simulink model "CtrPlatform_AdaptiveControl"  (Simulink 7.9)
settings: Solver=ode3  StartTime=0.0  StopTime=8  FixedStep=Ts  RelTol=1e-3
InitFcn:
  | eval('CtrPlatformCfg')
StopFcn:
  | eval('CtrPlotTrj')
values from neighbouring files (symbols this model uses):
  A = [a1 a2 a3 a4 a5 a6]/180*pi    [Config.m]    (also in CtrPlatformCfg.m)
  a2 = 0    [Config.m]    (also in CtrPlatformCfg.m)
  a3 = 0    [Config.m]    (also in CtrPlatformCfg.m)
  a4 = 0    [Config.m]    (also in CtrPlatformCfg.m)
  a5 = 90    [Config.m]    (also in CtrPlatformCfg.m)
  a6 = 0    [Config.m]    (also in CtrPlatformCfg.m)
  Cen = Cen(:)'    [Config.m]    (also in CtrPlatformCfg.m; DynEulerTest.m = Cen'; EfDynCAD.m = [cen1,cen2,cen3,cen4,cen5,cen6]')
  CurPulseFreq = 0.25*2*pi    (= 1.57079632679)    [Config.m]    (also in CtrPlatformCfg.m)
  Deg2Rad = pi/180    (= 0.0174532925199)    [Config.m]    (also in CtrPlatformCfg.m)
  DisturbSelect = 2    [Config.m]    (also in CtrPlatformCfg.m)
  DynTrjMode = 3    [Config.m]    (also in CtrPlatformCfg.m = 1)
  FbDisturbSelect = 2    [Config.m]    (also in CtrPlatformCfg.m)
  freq = tvel/radius    (= 1)    [Config.m]    (also in CtrPlatformCfg.m)
  FrictionSelect = 2    [CtrPlatformCfg.m]
  Gravity = 9.8    [Config.m]    (also in CtrPlatformCfg.m)
  Ie1 = in1(:)'    [Config.m]    (also in CtrPlatformCfg.m; DynEulerTest.m = in1(:); EfDynCAD.m = in1(:))
  Ie2 = in2(:)'    [Config.m]    (also in CtrPlatformCfg.m; DynEulerTest.m = in2(:); EfDynCAD.m = in2(:))
  Ie3 = in3(:)'    [Config.m]    (also in CtrPlatformCfg.m; DynEulerTest.m = in3(:); EfDynCAD.m = in3(:))
  Ie4 = in4(:)'    [Config.m]    (also in CtrPlatformCfg.m; DynEulerTest.m = in4(:); EfDynCAD.m = in4(:))
  Ie5 = in5(:)'    [Config.m]    (also in CtrPlatformCfg.m; DynEulerTest.m = in5(:); EfDynCAD.m = in5(:))
  Ie6 = in6(:)'    [Config.m]    (also in CtrPlatformCfg.m; DynEulerTest.m = in6(:); EfDynCAD.m = in6(:))
  in1 = [5.2954 -0.2565 -0.6366;-0.2565 4.7000 0.2830;-0.6366 0.2829 5.8635]    [Config.m]    (also in CtrPlatformCfg.m; DynEulerTest.m; EfDynCAD.m = [0.54  -0.01 0.23)
  in2 = [5.8840 0.0072 0.0135;0.0072 6.0178 -0.1907;0.0135 -0.1907 0.3374]    [Config.m]    (also in CtrPlatformCfg.m; DynEulerTest.m; EfDynCAD.m = (R_x*R_z)*in2*(R_x*R_z)')
  in3 = [1.8201 -0.2274 -0.3112;-0.2274 2.2537 -0.1441;-0.3112 -0.1441 1.9485]    [Config.m]    (also in CtrPlatformCfg.m; DynEulerTest.m; EfDynCAD.m = (R_x*R_z)*in3*(R_x*R_z)')
  in4 = [0.0607 -0.0922 0;-0.0922 1.4493 0;0 0 1.4620]    [Config.m]    (also in CtrPlatformCfg.m; DynEulerTest.m = [0.0607 -0.0922 0;-0.0922 1.4493 0;0 0,1.4620]; EfDynCAD.m = (R_y*Rz)*in4*(R_y*Rz)')
  in5 = [0.0191 0.0032 0;0.0032 0.0228 0;0 0 0.0291]    [Config.m]    (also in CtrPlatformCfg.m; DynEulerTest.m; EfDynCAD.m = (R_x*R_y)*in5*(R_x*R_y)')
  in6 = [0.0012 0 0;0 0.0007 0;0 0 0.0007]    [Config.m]    (also in CtrPlatformCfg.m; DynEulerTest.m; EfDynCAD.m = (R_y*Rz)*in6*(R_y*Rz)')
  init_Endx = gd_init(1,4)    [Config.m]    (also in CtrPlatformCfg.m)
  init_Endy = gd_init(2,4)    [Config.m]    (also in CtrPlatformCfg.m)
  init_Endz = gd_init(3,4)    [Config.m]    (also in CtrPlatformCfg.m)
  init_Rot = gd_init(1:3,1:3)    [Config.m]    (also in CtrPlatformCfg.m)
  InitialPos1 = A(1)*Rad2Line(1)    [CtrPlatformCfg.m]
  InitialPos2 = A(2)*Rad2Line(2)    [CtrPlatformCfg.m]
  InitialPos3 = A(3)*Rad2Line(3)    [CtrPlatformCfg.m]
  InitialPos4 = A(4)*Rad2Line(4)    [CtrPlatformCfg.m]
  InitialPos5 = A(5)*Rad2Line(5)    [CtrPlatformCfg.m]
  InitialPos6 = A(6)*Rad2Line(6)    [CtrPlatformCfg.m]
  JntOffset1 = A(1)    [Config.m]    (also in CtrPlatformCfg.m)
  JntOffset2 = A(2)    [Config.m]    (also in CtrPlatformCfg.m)
  JntOffset3 = A(3)    [Config.m]    (also in CtrPlatformCfg.m)
  JntOffset4 = A(4)    [Config.m]    (also in CtrPlatformCfg.m)
  JntOffset5 = A(5)    [Config.m]    (also in CtrPlatformCfg.m)
  JntOffset6 = A(6)    [Config.m]    (also in CtrPlatformCfg.m)
  L = [l1 l2 l3 l4 l5 l6 l7 l8 l9]    [Config.m]    (also in CtrPlatformCfg.m)
  LinePTs2RadpS = 2*pi/(EncRes*Ts)./Gear    [Config.m]    (also in CtrPlatformCfg.m)
  LinePTs2Rpm = 60/(EncRes*Ts)    (= 7.32421875)    [Config.m]    (also in CtrPlatformCfg.m)
  Ma = [ma1 ma2 ma3 ma4 ma5 ma6]    [Config.m]    (also in CtrPlatformCfg.m; DynEulerTest.m = [ma1; ma2; ma3; ma4; ma5; ma6]; EfDynCAD.m = [ma1 ma2 ma3 ma4 ma5 ma6]')
  ma1 = 170.31    [Config.m]    (also in CtrPlatformCfg.m; DynEulerTest.m; EfDynCAD.m = 77.75)
  ma2 = 63.74    [Config.m]    (also in CtrPlatformCfg.m; DynEulerTest.m; EfDynCAD.m = 32.31)
  ma3 = 98.98    [Config.m]    (also in CtrPlatformCfg.m; DynEulerTest.m; EfDynCAD.m = 18.61)
  ma4 = 24.46    [Config.m]    (also in CtrPlatformCfg.m; DynEulerTest.m; EfDynCAD.m = 15.65)
  ma5 = 5.24    [Config.m]    (also in CtrPlatformCfg.m; DynEulerTest.m; EfDynCAD.m = 3.32)
  ma6 = 0.6    [Config.m]    (also in CtrPlatformCfg.m; DynEulerTest.m; EfDynCAD.m)
  Pi0 = PiTest    [CtrPlatformCfg.m]
  PosPulseEnable = 1    [Config.m]    (also in CtrPlatformCfg.m)
  PosSourceSelect_Ad = 2    [CtrPlatformCfg.m]
  PosVelPulseGain = 500    [Config.m]    (also in CtrPlatformCfg.m)
  Rad2Line = Gear*EncRes/(2*pi)    [Config.m]    (also in CtrPlatformCfg.m)
  Rpm2LinePTs = EncRes*Ts/60    (= 0.136533333333)    [Config.m]    (also in CtrPlatformCfg.m)
  TrajSwitch = 1    [Config.m]    (also in CtrPlatformCfg.m)
  Trq2Cur = Trq2Cur./Cur2Trq    [Config.m]    (also in CtrPlatformCfg.m)
  Ts = 1/FrHz    (= 0.00025)    [Config.m]    (also in CtrPlatformCfg.m)
  Ts_Dyn = Ts    (= 0.00025)    [Config.m]    (also in CtrPlatformCfg.m)
  tvel = 120    [Config.m]    (also in CtrPlatformCfg.m)
  VelLpAxisNum = 1    [Config.m]    (also in CtrPlatformCfg.m)
  VelPulseEnable = 0    [Config.m]    (also in CtrPlatformCfg.m)
  VelPulseGain = 500    [Config.m]    (also in CtrPlatformCfg.m)
  Volt2Trq = Volt2Trq./Trq2Cur    [Config.m]    (also in CtrPlatformCfg.m)
undefined symbols (not defined in the file or in its folder): a1, DiscIntNeverNeededParam
libraries: simulink x56, mblibv1 x35, powerlib_extras x8, commnoisgen2 x2
(part 4 of 4)

== system CtrPlatform_AdaptiveControl/Friction Torque/Friction Torque/Ff2/Fp ==
  q : Inport
  Add : Sum  Inputs=++++  SampleTime=Ts
  B1 : Gain  Gain=B1  SampleTime=Ts
  B2 : Gain  Gain=B2  SampleTime=Ts
  B3 : Gain  Gain=B3  SampleTime=Ts
  B4 : Gain  Gain=B4  SampleTime=Ts
  Cosine : simulink/Lookup Tables/Cosine  Formula=cos(2*pi*u)  NumDataPoints=(2^5)+1  OutputWordLength=16
  Cosine1 : simulink/Lookup Tables/Cosine  Formula=cos(2*pi*u)  NumDataPoints=(2^5)+1  OutputWordLength=16
  Gain : Gain  Gain=1/(2*pi)  SampleTime=Ts
  Gain1 : Gain  Gain=1/pi  SampleTime=Ts
  Sine : simulink/Lookup Tables/Sine  Formula=sin(2*pi*u)  NumDataPoints=(2^5)+1  OutputWordLength=16
  Sine1 : simulink/Lookup Tables/Sine  Formula=sin(2*pi*u)  NumDataPoints=(2^5)+1  OutputWordLength=16
  Fp : Outport
  wires:
  Gain/1 -> Sine/1, Cosine/1
  Gain1/1 -> Sine1/1, Cosine1/1
  q/1 -> Gain/1, Gain1/1
  Cosine1/1 -> B4/1
  Sine1/1 -> B3/1
  Cosine/1 -> B2/1
  Sine/1 -> B1/1
  B2/1 -> Add/2
  B3/1 -> Add/3
  B4/1 -> Add/4
  B1/1 -> Add/1
  Add/1 -> Fp/1

== system CtrPlatform_AdaptiveControl/Friction Torque/Friction Torque/Ff2/Fv ==
  dq : Inport
  Abs : Abs  SampleTime=Ts
  Add : Sum  SampleTime=Ts
  Add1 : Sum  SampleTime=Ts
  Divide : Product  Inputs=*/  SampleTime=Ts
  Gain : Constant  Value=-1  SampleTime=Ts
  Math Function : Math  Operator=pow  SampleTime=Ts  SaturateOnIntegerOverflow=on
  Math Function1 : Math  SampleTime=Ts  SaturateOnIntegerOverflow=on
  Product{,1..3} (4 alike) : Product  SampleTime=Ts  RndMeth=Zero
  Sign : Signum  SampleTime=Ts
  Subtract : Sum  Inputs=-+  SampleTime=Ts
  dqs : Constant  Value=dqs  SampleTime=Ts
  fc : Constant  Value=fc  SampleTime=Ts
  fs : Constant  Value=fs  SampleTime=Ts
  lamda : Constant  Value=lamda  SampleTime=Ts
  theta : Constant  Value=theta  SampleTime=Ts
  Fv : Outport
  wires:
  dq/1 -> Divide/1, Sign/1, Product3/2
  dqs/1 -> Divide/2
  Divide/1 -> Abs/1
  Abs/1 -> Math Function/1
  lamda/1 -> Math Function/2
  Math Function/1 -> Product/1
  Gain/1 -> Product/2
  Product/1 -> Math Function1/1
  fc/1 -> Subtract/1, Add/1
  fs/1 -> Subtract/2
  Subtract/1 -> Product1/1
  Math Function1/1 -> Product1/2
  Product1/1 -> Add/2
  Sign/1 -> Product2/1
  Add/1 -> Product2/2
  Product3/1 -> Add1/1
  Product2/1 -> Add1/2
  theta/1 -> Product3/1
  Add1/1 -> Fv/1

== system CtrPlatform_AdaptiveControl/Friction Torque/Friction Torque/Ff3/Fp ==
  q : Inport
  Add : Sum  Inputs=++++  SampleTime=Ts
  B1 : Gain  Gain=B1  SampleTime=Ts
  B2 : Gain  Gain=B2  SampleTime=Ts
  B3 : Gain  Gain=B3  SampleTime=Ts
  B4 : Gain  Gain=B4  SampleTime=Ts
  Cosine : simulink/Lookup Tables/Cosine  Formula=cos(2*pi*u)  NumDataPoints=(2^5)+1  OutputWordLength=16
  Cosine1 : simulink/Lookup Tables/Cosine  Formula=cos(2*pi*u)  NumDataPoints=(2^5)+1  OutputWordLength=16
  Gain : Gain  Gain=1/(2*pi)  SampleTime=Ts
  Gain1 : Gain  Gain=1/pi  SampleTime=Ts
  Sine : simulink/Lookup Tables/Sine  Formula=sin(2*pi*u)  NumDataPoints=(2^5)+1  OutputWordLength=16
  Sine1 : simulink/Lookup Tables/Sine  Formula=sin(2*pi*u)  NumDataPoints=(2^5)+1  OutputWordLength=16
  Fp : Outport
  wires:
  Gain/1 -> Sine/1, Cosine/1
  Gain1/1 -> Sine1/1, Cosine1/1
  q/1 -> Gain/1, Gain1/1
  Cosine1/1 -> B4/1
  Sine1/1 -> B3/1
  Cosine/1 -> B2/1
  Sine/1 -> B1/1
  B2/1 -> Add/2
  B3/1 -> Add/3
  B4/1 -> Add/4
  B1/1 -> Add/1
  Add/1 -> Fp/1

== system CtrPlatform_AdaptiveControl/Friction Torque/Friction Torque/Ff3/Fv ==
  dq : Inport
  Abs : Abs  SampleTime=Ts
  Add : Sum  SampleTime=Ts
  Add1 : Sum  SampleTime=Ts
  Divide : Product  Inputs=*/  SampleTime=Ts
  Gain : Constant  Value=-1  SampleTime=Ts
  Math Function : Math  Operator=pow  SampleTime=Ts  SaturateOnIntegerOverflow=on
  Math Function1 : Math  SampleTime=Ts  SaturateOnIntegerOverflow=on
  Product{,1..3} (4 alike) : Product  SampleTime=Ts  RndMeth=Zero
  Sign : Signum  SampleTime=Ts
  Subtract : Sum  Inputs=-+  SampleTime=Ts
  dqs : Constant  Value=dqs  SampleTime=Ts
  fc : Constant  Value=fc  SampleTime=Ts
  fs : Constant  Value=fs  SampleTime=Ts
  lamda : Constant  Value=lamda  SampleTime=Ts
  theta : Constant  Value=theta  SampleTime=Ts
  Fv : Outport
  wires:
  dq/1 -> Divide/1, Sign/1, Product3/2
  dqs/1 -> Divide/2
  Divide/1 -> Abs/1
  Abs/1 -> Math Function/1
  lamda/1 -> Math Function/2
  Math Function/1 -> Product/1
  Gain/1 -> Product/2
  Product/1 -> Math Function1/1
  fc/1 -> Subtract/1, Add/1
  fs/1 -> Subtract/2
  Subtract/1 -> Product1/1
  Math Function1/1 -> Product1/2
  Product1/1 -> Add/2
  Sign/1 -> Product2/1
  Add/1 -> Product2/2
  Product3/1 -> Add1/1
  Product2/1 -> Add1/2
  theta/1 -> Product3/1
  Add1/1 -> Fv/1

== system CtrPlatform_AdaptiveControl/Friction Torque/Friction Torque/Ff4/Fp ==
  q : Inport
  Add : Sum  Inputs=++++  SampleTime=Ts
  B1 : Gain  Gain=B1  SampleTime=Ts
  B2 : Gain  Gain=B2  SampleTime=Ts
  B3 : Gain  Gain=B3  SampleTime=Ts
  B4 : Gain  Gain=B4  SampleTime=Ts
  Cosine : simulink/Lookup Tables/Cosine  Formula=cos(2*pi*u)  NumDataPoints=(2^5)+1  OutputWordLength=16
  Cosine1 : simulink/Lookup Tables/Cosine  Formula=cos(2*pi*u)  NumDataPoints=(2^5)+1  OutputWordLength=16
  Gain : Gain  Gain=1/(2*pi)  SampleTime=Ts
  Gain1 : Gain  Gain=1/pi  SampleTime=Ts
  Sine : simulink/Lookup Tables/Sine  Formula=sin(2*pi*u)  NumDataPoints=(2^5)+1  OutputWordLength=16
  Sine1 : simulink/Lookup Tables/Sine  Formula=sin(2*pi*u)  NumDataPoints=(2^5)+1  OutputWordLength=16
  Fp : Outport
  wires:
  Gain/1 -> Sine/1, Cosine/1
  Gain1/1 -> Sine1/1, Cosine1/1
  q/1 -> Gain/1, Gain1/1
  Cosine1/1 -> B4/1
  Sine1/1 -> B3/1
  Cosine/1 -> B2/1
  Sine/1 -> B1/1
  B2/1 -> Add/2
  B3/1 -> Add/3
  B4/1 -> Add/4
  B1/1 -> Add/1
  Add/1 -> Fp/1

== system CtrPlatform_AdaptiveControl/Friction Torque/Friction Torque/Ff4/Fv ==
  dq : Inport
  Abs : Abs  SampleTime=Ts
  Add : Sum  SampleTime=Ts
  Add1 : Sum  SampleTime=Ts
  Divide : Product  Inputs=*/  SampleTime=Ts
  Gain : Constant  Value=-1  SampleTime=Ts
  Math Function : Math  Operator=pow  SampleTime=Ts  SaturateOnIntegerOverflow=on
  Math Function1 : Math  SampleTime=Ts  SaturateOnIntegerOverflow=on
  Product{,1..3} (4 alike) : Product  SampleTime=Ts  RndMeth=Zero
  Sign : Signum  SampleTime=Ts
  Subtract : Sum  Inputs=-+  SampleTime=Ts
  dqs : Constant  Value=dqs  SampleTime=Ts
  fc : Constant  Value=fc  SampleTime=Ts
  fs : Constant  Value=fs  SampleTime=Ts
  lamda : Constant  Value=lamda  SampleTime=Ts
  theta : Constant  Value=theta  SampleTime=Ts
  Fv : Outport
  wires:
  dq/1 -> Divide/1, Sign/1, Product3/2
  dqs/1 -> Divide/2
  Divide/1 -> Abs/1
  Abs/1 -> Math Function/1
  lamda/1 -> Math Function/2
  Math Function/1 -> Product/1
  Gain/1 -> Product/2
  Product/1 -> Math Function1/1
  fc/1 -> Subtract/1, Add/1
  fs/1 -> Subtract/2
  Subtract/1 -> Product1/1
  Math Function1/1 -> Product1/2
  Product1/1 -> Add/2
  Sign/1 -> Product2/1
  Add/1 -> Product2/2
  Product3/1 -> Add1/1
  Product2/1 -> Add1/2
  theta/1 -> Product3/1
  Add1/1 -> Fv/1

== system CtrPlatform_AdaptiveControl/Friction Torque/Friction Torque/Ff5/Fp ==
  q : Inport
  Add : Sum  Inputs=++++  SampleTime=Ts
  B1 : Gain  Gain=B1  SampleTime=Ts
  B2 : Gain  Gain=B2  SampleTime=Ts
  B3 : Gain  Gain=B3  SampleTime=Ts
  B4 : Gain  Gain=B4  SampleTime=Ts
  Cosine : simulink/Lookup Tables/Cosine  Formula=cos(2*pi*u)  NumDataPoints=(2^5)+1  OutputWordLength=16
  Cosine1 : simulink/Lookup Tables/Cosine  Formula=cos(2*pi*u)  NumDataPoints=(2^5)+1  OutputWordLength=16
  Gain : Gain  Gain=1/(2*pi)  SampleTime=Ts
  Gain1 : Gain  Gain=1/pi  SampleTime=Ts
  Sine : simulink/Lookup Tables/Sine  Formula=sin(2*pi*u)  NumDataPoints=(2^5)+1  OutputWordLength=16
  Sine1 : simulink/Lookup Tables/Sine  Formula=sin(2*pi*u)  NumDataPoints=(2^5)+1  OutputWordLength=16
  Fp : Outport
  wires:
  Gain/1 -> Sine/1, Cosine/1
  Gain1/1 -> Sine1/1, Cosine1/1
  q/1 -> Gain/1, Gain1/1
  Cosine1/1 -> B4/1
  Sine1/1 -> B3/1
  Cosine/1 -> B2/1
  Sine/1 -> B1/1
  B2/1 -> Add/2
  B3/1 -> Add/3
  B4/1 -> Add/4
  B1/1 -> Add/1
  Add/1 -> Fp/1

== system CtrPlatform_AdaptiveControl/Friction Torque/Friction Torque/Ff5/Fv ==
  dq : Inport
  Abs : Abs  SampleTime=Ts
  Add : Sum  SampleTime=Ts
  Add1 : Sum  SampleTime=Ts
  Divide : Product  Inputs=*/  SampleTime=Ts
  Gain : Constant  Value=-1  SampleTime=Ts
  Math Function : Math  Operator=pow  SampleTime=Ts  SaturateOnIntegerOverflow=on
  Math Function1 : Math  SampleTime=Ts  SaturateOnIntegerOverflow=on
  Product{,1..3} (4 alike) : Product  SampleTime=Ts  RndMeth=Zero
  Sign : Signum  SampleTime=Ts
  Subtract : Sum  Inputs=-+  SampleTime=Ts
  dqs : Constant  Value=dqs  SampleTime=Ts
  fc : Constant  Value=fc  SampleTime=Ts
  fs : Constant  Value=fs  SampleTime=Ts
  lamda : Constant  Value=lamda  SampleTime=Ts
  theta : Constant  Value=theta  SampleTime=Ts
  Fv : Outport
  wires:
  dq/1 -> Divide/1, Sign/1, Product3/2
  dqs/1 -> Divide/2
  Divide/1 -> Abs/1
  Abs/1 -> Math Function/1
  lamda/1 -> Math Function/2
  Math Function/1 -> Product/1
  Gain/1 -> Product/2
  Product/1 -> Math Function1/1
  fc/1 -> Subtract/1, Add/1
  fs/1 -> Subtract/2
  Subtract/1 -> Product1/1
  Math Function1/1 -> Product1/2
  Product1/1 -> Add/2
  Sign/1 -> Product2/1
  Add/1 -> Product2/2
  Product3/1 -> Add1/1
  Product2/1 -> Add1/2
  theta/1 -> Product3/1
  Add1/1 -> Fv/1

== system CtrPlatform_AdaptiveControl/Friction Torque/Friction Torque/Ff6/Fp ==
  q : Inport
  Add : Sum  Inputs=++++  SampleTime=Ts
  B1 : Gain  Gain=B1  SampleTime=Ts
  B2 : Gain  Gain=B2  SampleTime=Ts
  B3 : Gain  Gain=B3  SampleTime=Ts
  B4 : Gain  Gain=B4  SampleTime=Ts
  Cosine : simulink/Lookup Tables/Cosine  Formula=cos(2*pi*u)  NumDataPoints=(2^5)+1  OutputWordLength=16
  Cosine1 : simulink/Lookup Tables/Cosine  Formula=cos(2*pi*u)  NumDataPoints=(2^5)+1  OutputWordLength=16
  Gain : Gain  Gain=1/(2*pi)  SampleTime=Ts
  Gain1 : Gain  Gain=1/pi  SampleTime=Ts
  Sine : simulink/Lookup Tables/Sine  Formula=sin(2*pi*u)  NumDataPoints=(2^5)+1  OutputWordLength=16
  Sine1 : simulink/Lookup Tables/Sine  Formula=sin(2*pi*u)  NumDataPoints=(2^5)+1  OutputWordLength=16
  Fp : Outport
  wires:
  Gain/1 -> Sine/1, Cosine/1
  Gain1/1 -> Sine1/1, Cosine1/1
  q/1 -> Gain/1, Gain1/1
  Cosine1/1 -> B4/1
  Sine1/1 -> B3/1
  Cosine/1 -> B2/1
  Sine/1 -> B1/1
  B2/1 -> Add/2
  B3/1 -> Add/3
  B4/1 -> Add/4
  B1/1 -> Add/1
  Add/1 -> Fp/1

== system CtrPlatform_AdaptiveControl/Friction Torque/Friction Torque/Ff6/Fv ==
  dq : Inport
  Abs : Abs  SampleTime=Ts
  Add : Sum  SampleTime=Ts
  Add1 : Sum  SampleTime=Ts
  Divide : Product  Inputs=*/  SampleTime=Ts
  Gain : Constant  Value=-1  SampleTime=Ts
  Math Function : Math  Operator=pow  SampleTime=Ts  SaturateOnIntegerOverflow=on
  Math Function1 : Math  SampleTime=Ts  SaturateOnIntegerOverflow=on
  Product{,1..3} (4 alike) : Product  SampleTime=Ts  RndMeth=Zero
  Sign : Signum  SampleTime=Ts
  Subtract : Sum  Inputs=-+  SampleTime=Ts
  dqs : Constant  Value=dqs  SampleTime=Ts
  fc : Constant  Value=fc  SampleTime=Ts
  fs : Constant  Value=fs  SampleTime=Ts
  lamda : Constant  Value=lamda  SampleTime=Ts
  theta : Constant  Value=theta  SampleTime=Ts
  Fv : Outport
  wires:
  dq/1 -> Divide/1, Sign/1, Product3/2
  dqs/1 -> Divide/2
  Divide/1 -> Abs/1
  Abs/1 -> Math Function/1
  lamda/1 -> Math Function/2
  Math Function/1 -> Product/1
  Gain/1 -> Product/2
  Product/1 -> Math Function1/1
  fc/1 -> Subtract/1, Add/1
  fs/1 -> Subtract/2
  Subtract/1 -> Product1/1
  Math Function1/1 -> Product1/2
  Product1/1 -> Add/2
  Sign/1 -> Product2/1
  Add/1 -> Product2/2
  Product3/1 -> Add1/1
  Product2/1 -> Add1/2
  theta/1 -> Product3/1
  Add1/1 -> Fv/1

== matlab function Trajectory Generator/Still/Inverse Kinematic ==
  data: EndPos input double; init_Rot parameter double; Theta output double; L parameter double
function Theta = fcn(EndPos,init_Rot,L)
%#eml
Theta =[0;0; 0; 0; 0; 0];
gd = [init_Rot,EndPos;[0 0 0],1];
[Theta_total,num_total] = inv_kin(gd,L);
%%%%%%%%%%%Need to modify%%%%%%%%%%%%%%%
Theta = Theta_total(:,2);

== matlab function Trajectory Generator/Still/Jacobian ==
  data: Theta input double; Omega output double; EndVel input double; L parameter double
function Omega = fcn(Theta,EndVel,L)
%#eml

Omega = zeros(6,1);
V = [EndVel; 0; 0; 0];   
g = fwd_kin(L,Theta');
Jb = body_Jacobian(L,Theta');
Adg_inv = double(AdjointInv(g));
Omega = double((Jb \ Adg_inv* V)')';

== matlab function Dynamics/M*Acc ==
  data: RefAcc input double; EnTheta input double; M_Acc output double; L parameter double; Cen parameter double; Ma parameter double; Ie1 parameter double; Ie2 parameter double; Ie3 parameter double; Ie4 parameter double; Ie5 parameter double; Ie6 parameter double
function M_Acc = fcn(RefAcc,EnTheta,L,Cen,Ma,Ie1,Ie2,Ie3,Ie4,Ie5,Ie6)
%#eml

M_Acc = zeros(6,1);
M_Acc = M_d(L/1000,EnTheta',Cen,Ma,Ie1,Ie2,Ie3,Ie4,Ie5,Ie6)*RefAcc;

== matlab function Dynamics/C*Omega ==
  data: RefOmega input double; C_Omega output double; EnTheta input double; EnOmega input double; L parameter double; Cen parameter double; Ma parameter double; Ie1 parameter double; Ie2 parameter double; Ie3 parameter double; Ie4 parameter double; Ie5 parameter double; Ie6 parameter double
function C_Omega = fcn(RefOmega,EnTheta,EnOmega,L,Cen,Ma,Ie1,Ie2,Ie3,Ie4,Ie5,Ie6)
%#eml

C_Omega =zeros(6,1);

L=L/1000;
M_dp = zeros(6,6*6);
M_dp(:,1:6) = M_dp1(L,EnTheta',Cen,Ma,Ie1,Ie2,Ie3,Ie4,Ie5,Ie6);
M_dp(:,7:12) = M_dp2(L,EnTheta',Cen,Ma,Ie1,Ie2,Ie3,Ie4,Ie5,Ie6);
M_dp(:,13:18) = M_dp3(L,EnTheta',Cen,Ma,Ie1,Ie2,Ie3,Ie4,Ie5,Ie6);
M_dp(:,19:24)= M_dp4(L,EnTheta',Cen,Ma,Ie1,Ie2,Ie3,Ie4,Ie5,Ie6);
M_dp(:,25:30) = M_dp5(L,EnTheta',Cen,Ma,Ie1,Ie2,Ie3,Ie4,Ie5,Ie6);
M_dp(:,31:36) = M_dp6(L,EnTheta',Cen,Ma,Ie1,Ie2,Ie3,Ie4,Ie5,Ie6);

C = zeros(6,6);

for i=1:6
    for j=1:6
        for k=1:6
                 C(i,j) =C(i,j)+ 0.5*(M_dp(i,(k-1)*6+j)+M_dp(i,(j-1)*6+k)-M_dp(k,(i-1)*6+j))*EnOmega(k);
            
        end
    end
end
C_Omega = C*RefOmega;
% end

== matlab function Dynamics/N ==
  data: EnTheta input double; N output double; L parameter double; Cen parameter double; Ma parameter double; Gravity parameter double
function N = fcn(EnTheta,L,Cen,Ma,Gravity)
%#eml
N=zeros(6,1);
N=N_d(L/1000,EnTheta',Cen,Ma,Gravity);

== matlab function Trajectory Generator/Circle in Descartes Space/Inverse Kinematic ==
  data: EndPos input double; init_Rot parameter double; Theta output double; L parameter double
function Theta = fcn(EndPos,init_Rot,L)
%#eml
Theta =[0;0; 0; 0; 0; 0];
gd = [init_Rot,EndPos;[0 0 0],1];
[Theta_total,num_total] = inv_kin(gd,L);
%%%%%%%%%%%Need to modify%%%%%%%%%%%%%%%
Theta = Theta_total(:,2);

== matlab function Trajectory Generator/Circle in Descartes Space/Jacobian ==
  data: Theta input double; Omega output double; EndVel input double; L parameter double
function Omega = fcn(Theta,EndVel,L)
%#eml

Omega = zeros(6,1);
V = [EndVel; 0; 0; 0];   
g = fwd_kin(L,Theta');
Jb = body_Jacobian(L,Theta');
Adg_inv = double(AdjointInv(g));
Omega = double((Jb \ Adg_inv* V)')';

== matlab function Controller/MATLAB Function ==
  data: qr2 input double; qr1 input double; q input double; Y output double
function Y = fcn(qr2,qr1,q)
%#codegen
gr=9.8;
l1 = 566;
l2 = 150;
l3 = 870;
l4 = 170;
l5 = 1016;
l6 = 154;
l7 = 20;
l8 = 0;
l9 = 0;
Ld=[l1 l2 l3 l4 l5]/1000;
q=q';
qr1=qr1';
qr2=qr2';
Y=EulerWd_Min(Ld,q,qr1,qr2,gr);
end

== matlab function Controller/MATLAB Function1 ==
  data: Y input double; sigma input double; Kpi input double; py1 output double
function py1 = fcn(Y,sigma,Kpi)
%#codegen
py1=inv(Kpi)*Y'*sigma;
end

== matlab function Trajectory Generator/Line in Joint Space/Forward ==
  data: Theta input double; EndPos output double; L parameter double
function EndPos = fcn(Theta,L)
%#eml
gd = fwd_kin(L,Theta');
EndPos = gd(1:3,4);

== matlab function Trajectory Generator/Line in Joint Space/Jacobian ==
  data: Theta input double; Omega input double; EndVel output double; L parameter double
function EndVel = fcn(Theta,Omega,L)
%#eml


EndVW = spat_Jacobian(L,Theta')*Omega;
gd = fwd_kin(L,Theta');
EndW = EndVW(4:6,1);
gd_pos = gd(1:3,4);
EndVel=cross(EndW,gd_pos);
